simulink model "practica7_simulink"  (R2024b)
settings: Solver=VariableStepAuto  StartTime=0.0  StopTime=10  RelTol=1e-3
values from neighbouring files (symbols this model uses):
  R2 = 5e6    (= 5000000)    [OPAM_practica7.m]
undefined symbols (not defined in the file or in its folder): op1, op2

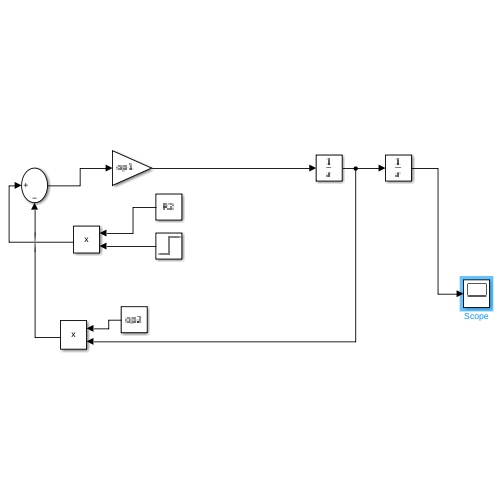
[thumbnail: Simulink's stored preview of the top-level diagram]
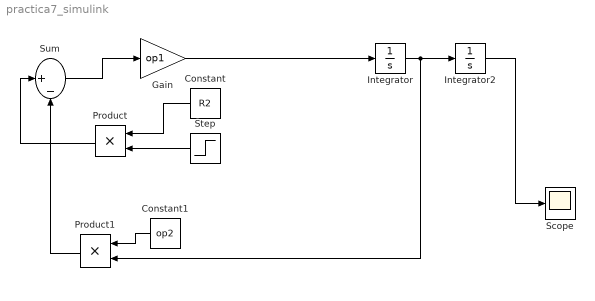
== system practica7_simulink ==
  Constant : Constant  Value=R2
  Constant1 : Constant  Value=op2
  Gain : Gain  Gain=op1
  Integrator : Integrator
  Integrator2 : Integrator
  Product : Product
  Product1 : Product
  Scope : Scope
  Step : Step  Time=0  After=12  SampleTime=0
  Sum : Sum  Inputs=|+-
  wires:
  Gain/1 -> Integrator/1
  Constant/1 -> Product/1
  Product/1 -> Sum/1
  Product1/1 -> Sum/2
  Sum/1 -> Gain/1
  Step/1 -> Product/2
  Constant1/1 -> Product1/1
  Integrator/1 -> Product1/2, Integrator2/1
  Integrator2/1 -> Scope/1
